simulink model "DFADAS2_SenFus_v1_201204RC_training_210115"  (R2018b)
settings: Solver=FixedStepDiscrete  StartTime=0.0  StopTime=inf  FixedStep=0.002  RelTol=1e-3  EnableMultiTasking=on
PreLoadFcn:
  | RTWConfigurationCB('preloadfcn', bdroot);
libraries: canmsglib x108, simulink x48, canfdmsglib x12
(part 19 of 28)

== system DFADAS2_SenFus_v1_201204RC_training_210115/Signal Input (Input)/Signal Input (50ms) (Input50)/Rear Right Radar(S1) Objects Information (RRRdr)/S0 Data Frame Read/Enabled Subsystem/M2ObjInfo/Subsystem1 ==
  const : Inport
  RemainderCnt : Inport  Port=2
  In : Inport  Port=3
  If : If  IfExpression=u1 >=0
  If Action Subsystem : Subsystem  TreatAsAtomicUnit=on
  If Action Subsystem1 : Subsystem  TreatAsAtomicUnit=on
  Merge : Merge
  Out : Outport
  wires:
  In/1 -> If Action Subsystem1/1(In1)
  const/1 -> If/1
  If/1 -> If Action Subsystem/Action
  If Action Subsystem1/1(Out1) -> Merge/2
  If/2 -> If Action Subsystem1/Action
  Merge/1 -> Out/1
  If Action Subsystem/1(Out1) -> Merge/1

== system DFADAS2_SenFus_v1_201204RC_training_210115/Signal Input (Input)/Signal Input (50ms) (Input50)/Rear Right Radar(S1) Objects Information (RRRdr)/S0 Data Frame Read/Enabled Subsystem/M3ObjInfo/If Action Subsystem1 ==
  msg : Inport
  "MValueSel " : Inport  Port=2
  obj_num : Inport  Port=3
  Action Port : ActionPort  ActionType=then
  Add : Sum
  Add2 : Sum
  Gain : Gain  Gain=48
  MValueSel : Constant  Value=24
  MValueSel2 : Constant  Value=[1:24]
  Product : Product
  Scope3 : Scope
  Selector : Selector  InputPortWidth=240  IndexOptions=Index vector (port)  Indices=[1 3]  OutputSizes=1
  Selector1 : Selector  InputPortWidth=240  IndexOptions=Index vector (port)  Indices=[1 3]  OutputSizes=1
  M30ObjInfo : Outport
  M31ObjInfo : Outport  Port=2
  wires:
  Product/1 -> M31ObjInfo/1
  obj_num/1 -> Scope3/1, Product/2
  Selector1/1 -> Product/1
  "MValueSel "/1 -> Gain/1
  Gain/1 -> Add2/1
  msg/1 -> Selector1/1, Selector/1
  Add/1 -> Selector1/2
  MValueSel/1 -> Add/2
  Add2/1 -> Selector/2, Add/1
  MValueSel2/1 -> Add2/2
  Selector/1 -> M30ObjInfo/1

== system DFADAS2_SenFus_v1_201204RC_training_210115/Signal Input (Input)/Signal Input (50ms) (Input50)/Rear Right Radar(S1) Objects Information (RRRdr)/S0 Data Frame Read/Enabled Subsystem/M3ObjInfo/If Action Subsystem2 ==
  Action Port : ActionPort  ActionType=elseif
  Constant : Constant  Value=[0 0 0 0 0 0 0 0 0 0 0 0 0 0 0 0 0 0 0 0 0 0 0 0]
  Constant1 : Constant  Value=[0 0 0 0 0 0 0 0 0 0 0 0 0 0 0 0 0 0 0 0 0 0 0 0]
  ZeroObjInfo0 : Outport
  ZeroObjInfo1 : Outport  Port=2
  wires:
  Constant/1 -> ZeroObjInfo0/1
  Constant1/1 -> ZeroObjInfo1/1

== system DFADAS2_SenFus_v1_201204RC_training_210115/Signal Input (Input)/Signal Input (50ms) (Input50)/Rear Right Radar(S1) Objects Information (RRRdr)/S0 Data Frame Read/Enabled Subsystem/M3ObjInfo/Subsystem1 ==
  const : Inport
  RemainderCnt : Inport  Port=2
  In : Inport  Port=3
  If : If  IfExpression=u1 >=0
  If Action Subsystem : Subsystem  TreatAsAtomicUnit=on
  If Action Subsystem1 : Subsystem  TreatAsAtomicUnit=on
  Merge : Merge
  Out : Outport
  wires:
  In/1 -> If Action Subsystem1/1(In1)
  const/1 -> If/1
  If/1 -> If Action Subsystem/Action
  If Action Subsystem1/1(Out1) -> Merge/2
  If/2 -> If Action Subsystem1/Action
  Merge/1 -> Out/1
  If Action Subsystem/1(Out1) -> Merge/1

== system DFADAS2_SenFus_v1_201204RC_training_210115/Signal Input (Input)/Signal Input (50ms) (Input50)/Rear Right Radar(S1) Objects Information (RRRdr)/S0 Data Frame Read/Enabled Subsystem/M4ObjInfo1/If Action Subsystem1 ==
  msg : Inport
  "MValueSel " : Inport  Port=2
  "obj_num " : Inport  Port=3
  Action Port : ActionPort  ActionType=then
  Add : Sum
  Add2 : Sum
  Gain : Gain  Gain=48
  MValueSel : Constant  Value=24
  MValueSel2 : Constant  Value=[1:24]
  Product : Product
  Scope3 : Scope
  Selector : Selector  InputPortWidth=240  IndexOptions=Index vector (port)  Indices=[1 3]  OutputSizes=1
  Selector1 : Selector  InputPortWidth=240  IndexOptions=Index vector (port)  Indices=[1 3]  OutputSizes=1
  M40ObjInfo : Outport
  M41ObjInfo : Outport  Port=2
  wires:
  Product/1 -> M41ObjInfo/1
  "obj_num "/1 -> Scope3/1, Product/2
  Selector1/1 -> Product/1
  Selector/1 -> M40ObjInfo/1
  MValueSel2/1 -> Add2/2
  Add2/1 -> Add/1, Selector/2
  MValueSel/1 -> Add/2
  Add/1 -> Selector1/2
  msg/1 -> Selector/1, Selector1/1
  Gain/1 -> Add2/1
  "MValueSel "/1 -> Gain/1

== system DFADAS2_SenFus_v1_201204RC_training_210115/Signal Input (Input)/Signal Input (50ms) (Input50)/Rear Right Radar(S1) Objects Information (RRRdr)/S0 Data Frame Read/Enabled Subsystem/M4ObjInfo1/If Action Subsystem2 ==
  Action Port : ActionPort  ActionType=elseif
  Constant : Constant  Value=[0 0 0 0 0 0 0 0 0 0 0 0 0 0 0 0 0 0 0 0 0 0 0 0]
  Constant1 : Constant  Value=[0 0 0 0 0 0 0 0 0 0 0 0 0 0 0 0 0 0 0 0 0 0 0 0]
  ZeroObjInfo0 : Outport
  ZeroObjInfo1 : Outport  Port=2
  wires:
  Constant1/1 -> ZeroObjInfo1/1
  Constant/1 -> ZeroObjInfo0/1

== system DFADAS2_SenFus_v1_201204RC_training_210115/Signal Input (Input)/Signal Input (50ms) (Input50)/Rear Right Radar(S1) Objects Information (RRRdr)/S0 Data Frame Read/Enabled Subsystem/M4ObjInfo1/Subsystem1 ==
  const : Inport
  RemainderCnt : Inport  Port=2
  In : Inport  Port=3
  If : If  IfExpression=u1 >=0
  If Action Subsystem : Subsystem  TreatAsAtomicUnit=on
  If Action Subsystem1 : Subsystem  TreatAsAtomicUnit=on
  Merge : Merge
  Out : Outport
  wires:
  In/1 -> If Action Subsystem1/1(In1)
  const/1 -> If/1
  If/1 -> If Action Subsystem/Action
  If Action Subsystem1/1(Out1) -> Merge/2
  If/2 -> If Action Subsystem1/Action
  Merge/1 -> Out/1
  If Action Subsystem/1(Out1) -> Merge/1

== system DFADAS2_SenFus_v1_201204RC_training_210115/Signal Input (Input)/Signal Input (50ms) (Input50)/Rear Right Radar(S1) Objects Information (RRRdr)/S0 Data Frame Read/Enabled Subsystem/Unpack/If Action Subsystem ==
  msg : Inport
  Action Port : ActionPort  ActionType=then
  Unpack : Subsystem
  RLRdrObjInfo : Outport
  MValue : Outport  Port=2
  wires:
  Unpack/1(RRRdrObjInfo) -> RLRdrObjInfo/1
  msg/1 -> Unpack/1(msg)
  Unpack/2(MValue) -> MValue/1

== system DFADAS2_SenFus_v1_201204RC_training_210115/Signal Input (Input)/Signal Input (50ms) (Input50)/Rear Right Radar(S1) Objects Information (RRRdr)/S0 Data Frame Read/Enabled Subsystem/Unpack/If Action Subsystem1 ==
  Action Port : ActionPort  ActionType=elseif
  Constant : Constant  Value=99
  DflMValue : Outport
  wires:
  Constant/1 -> DflMValue/1

== system DFADAS2_SenFus_v1_201204RC_training_210115/Signal Input (Input)/Signal Input (10ms) (Input10)/VehInfo/Body Electric System State Receive and Processing (BESRx)/Steering Lamp CAN Frame PreProcess (StLampCANFrmPPrcs)/CAN Diagnosis (CANDia)/CheckSum Diagnosis (ChkSumDia)/Bit Check(BChk) ==
  note: Bit Check Discription:
      | Byte0: Checksum
      | Byte1-7: Test signal
  BChk_bRawDa : Inport
  Bit Operating (BOp) : Subsystem
  Byte0 : Selector  IndexMode=Zero-based  InputPortWidth=8  IndexOptions=Index vector (dialog)  Indices=0  OutputSizes=1
  Byte1 : Selector  IndexMode=Zero-based  InputPortWidth=8  IndexOptions=Index vector (dialog)  Indices=1  OutputSizes=1
  Byte2 : Selector  IndexMode=Zero-based  InputPortWidth=8  IndexOptions=Index vector (dialog)  Indices=2  OutputSizes=1
  Byte3 : Selector  IndexMode=Zero-based  InputPortWidth=8  IndexOptions=Index vector (dialog)  Indices=3  OutputSizes=1
  Byte4 : Selector  IndexMode=Zero-based  InputPortWidth=8  IndexOptions=Index vector (dialog)  Indices=4  OutputSizes=1
  Byte5 : Selector  IndexMode=Zero-based  InputPortWidth=8  IndexOptions=Index vector (dialog)  Indices=5  OutputSizes=1
  Byte6 : Selector  IndexMode=Zero-based  InputPortWidth=8  IndexOptions=Index vector (dialog)  Indices=6  OutputSizes=1
  Byte7 : Selector  IndexMode=Zero-based  InputPortWidth=8  IndexOptions=Index vector (dialog)  Indices=7  OutputSizes=1
  BChk_efErrFlg : Outport
  wires:
  Byte0/1 -> Bit Operating (BOp)/1(BOp_bByte0)
  Bit Operating (BOp)/1(BOp_efChkSumErrFlg) -> BChk_efErrFlg/1
  Byte7/1 -> Bit Operating (BOp)/8(BOp_bByte7)
  Byte6/1 -> Bit Operating (BOp)/7(BOp_bByte6)
  Byte5/1 -> Bit Operating (BOp)/6(BOp_bByte5)
  Byte4/1 -> Bit Operating (BOp)/5(BOp_bByte4)
  Byte3/1 -> Bit Operating (BOp)/4(BOp_bByte3)
  Byte2/1 -> Bit Operating (BOp)/3(BOp_bByte2)
  Byte1/1 -> Bit Operating (BOp)/2(BOp_bByte1)
  BChk_bRawDa/1 -> Byte7/1, Byte6/1, Byte5/1, Byte4/1, Byte3/1, Byte2/1, Byte1/1, Byte0/1

== system DFADAS2_SenFus_v1_201204RC_training_210115/Signal Input (Input)/Signal Input (10ms) (Input10)/VehInfo/Function Keys State Receive and Processing (FKeyStRx)/Key Enable CAN Frame PreProcess (KeyEnaCANFrmPPrcs)/CAN Diagnosis (CANDia)/CheckSum Diagnosis (ChkSumDia)/Bit Check(BChk) ==
  note: Bit Check Discription:
      | Byte0: Checksum
      | Byte1-7: Test signal
  BChk_bRawDa : Inport
  Bit Operating (BOp) : Subsystem
  Byte0 : Selector  IndexMode=Zero-based  InputPortWidth=8  IndexOptions=Index vector (dialog)  Indices=0  OutputSizes=1
  Byte1 : Selector  IndexMode=Zero-based  InputPortWidth=8  IndexOptions=Index vector (dialog)  Indices=1  OutputSizes=1
  Byte2 : Selector  IndexMode=Zero-based  InputPortWidth=8  IndexOptions=Index vector (dialog)  Indices=2  OutputSizes=1
  Byte3 : Selector  IndexMode=Zero-based  InputPortWidth=8  IndexOptions=Index vector (dialog)  Indices=3  OutputSizes=1
  Byte4 : Selector  IndexMode=Zero-based  InputPortWidth=8  IndexOptions=Index vector (dialog)  Indices=4  OutputSizes=1
  Byte5 : Selector  IndexMode=Zero-based  InputPortWidth=8  IndexOptions=Index vector (dialog)  Indices=5  OutputSizes=1
  Byte6 : Selector  IndexMode=Zero-based  InputPortWidth=8  IndexOptions=Index vector (dialog)  Indices=6  OutputSizes=1
  Byte7 : Selector  IndexMode=Zero-based  InputPortWidth=8  IndexOptions=Index vector (dialog)  Indices=7  OutputSizes=1
  BChk_efErrFlg : Outport
  wires:
  BChk_bRawDa/1 -> Byte0/1, Byte1/1, Byte2/1, Byte3/1, Byte4/1, Byte5/1, Byte6/1, Byte7/1
  Byte1/1 -> Bit Operating (BOp)/2(BOp_bByte1)
  Byte2/1 -> Bit Operating (BOp)/3(BOp_bByte2)
  Byte3/1 -> Bit Operating (BOp)/4(BOp_bByte3)
  Byte4/1 -> Bit Operating (BOp)/5(BOp_bByte4)
  Byte5/1 -> Bit Operating (BOp)/6(BOp_bByte5)
  Byte6/1 -> Bit Operating (BOp)/7(BOp_bByte6)
  Byte7/1 -> Bit Operating (BOp)/8(BOp_bByte7)
  Bit Operating (BOp)/1(BOp_efChkSumErrFlg) -> BChk_efErrFlg/1
  Byte0/1 -> Bit Operating (BOp)/1(BOp_bByte0)

== system DFADAS2_SenFus_v1_201204RC_training_210115/Signal Input (Input)/Signal Input (10ms) (Input10)/VehInfo/MP5 Signal Receive (MP5Rx)1/CAN Diagnosis (CANDia)/CheckSum Diagnosis (ChkSumDia)/Bit Check(BChk)/Bit Operating (BOp) ==
  note: CheckSum Error Flag Discription:
      | 1 : Fault
      | 0 : Normal
  note: Checksum Preprocess -- ChksumPre
  Chksum in Frame : Inport
  BOp_bByte1 : Inport  Port=2
  BOp_bByte2 : Inport  Port=3
  BOp_bByte3 : Inport  Port=4
  BOp_bByte4 : Inport  Port=5
  BOp_bByte5 : Inport  Port=6
  BOp_bByte6 : Inport  Port=7
  BOp_bByte7 : Inport  Port=8
  Add : Sum  Inputs=+++++++
  Add1 : Sum  Inputs=+-
  Add2 : Sum  Inputs=+-
  ChksumPre1 : Subsystem
  ChksumPre2 : Subsystem
  ChksumPre3 : Subsystem
  ChksumPre4 : Subsystem
  ChksumPre5 : Subsystem
  ChksumPre6 : Subsystem
  ChksumPre7 : Subsystem
  Constant : Constant  Value=256  OutDataTypeStr=uint16  SampleTime=-1
  Constant1 : Constant  Value=255  OutDataTypeStr=uint8  SampleTime=-1
  Constant2 : Constant  OutDataTypeStr=uint8  SampleTime=-1
  Constant3 : Constant  Value=0  OutDataTypeStr=uint8  SampleTime=-1
  Data Type Conversion6 : DataTypeConversion  OutDataTypeStr=uint8
  Math Function : Math  Operator=mod  OutputSignalType=real  SaturateOnIntegerOverflow=on
  Switch : Switch  Criteria=u2 ~= 0
  BOp_efChkSumErrFlg : Outport
  wires:
  Switch/1 -> BOp_efChkSumErrFlg/1
  Constant3/1 -> Switch/3
  Constant2/1 -> Switch/1
  BOp_bByte7/1 -> ChksumPre7/1(In1)
  ChksumPre7/1(Out1) -> Add/7
  ChksumPre6/1(Out1) -> Add/6
  BOp_bByte6/1 -> ChksumPre6/2(In2)
  BOp_bByte5/1 -> ChksumPre6/1(In1)
  ChksumPre5/1(Out1) -> Add/5
  BOp_bByte4/1 -> ChksumPre5/2(In2)
  BOp_bByte3/1 -> ChksumPre5/1(In1)
  ChksumPre4/1(Out1) -> Add/4
  BOp_bByte2/1 -> ChksumPre4/1(In1), ChksumPre3/1(In1), ChksumPre2/1(In1)
  ChksumPre1/1(Out1) -> Add/1
  BOp_bByte1/1 -> ChksumPre1/1(In1)
  Constant1/1 -> Add1/1
  Math Function/1 -> Data Type Conversion6/1
  Constant/1 -> Math Function/2
  Add/1 -> Math Function/1
  Data Type Conversion6/1 -> Add1/2
  ChksumPre2/1(Out1) -> Add/2
  ChksumPre3/1(Out1) -> Add/3
  Chksum in Frame/1 -> Add2/1
  Add1/1 -> Add2/2
  Add2/1 -> Switch/2

== system DFADAS2_SenFus_v1_201204RC_training_210115/Signal Input (Input)/Signal Input (10ms) (Input10)/VehInfo/Vehicle Movement Signal Receive and Processing (VehMovRx)/VehSpd CAN Frame PreProcess (VehSpdCANFrmPPrcs)/CAN Diagnosis (CANDia)/CheckSum Diagnosis (ChkSumDia)/Bit Check(BChk) ==
  note: Bit Check Discription:
      | Byte0: Checksum
      | Byte1-7: Test signal
  BChk_bRawDa : Inport
  Bit Operating (BOp) : Subsystem
  Byte0 : Selector  IndexMode=Zero-based  InputPortWidth=8  IndexOptions=Index vector (dialog)  Indices=0  OutputSizes=1
  Byte1 : Selector  IndexMode=Zero-based  InputPortWidth=8  IndexOptions=Index vector (dialog)  Indices=1  OutputSizes=1
  Byte2 : Selector  IndexMode=Zero-based  InputPortWidth=8  IndexOptions=Index vector (dialog)  Indices=2  OutputSizes=1
  Byte3 : Selector  IndexMode=Zero-based  InputPortWidth=8  IndexOptions=Index vector (dialog)  Indices=3  OutputSizes=1
  Byte4 : Selector  IndexMode=Zero-based  InputPortWidth=8  IndexOptions=Index vector (dialog)  Indices=4  OutputSizes=1
  Byte5 : Selector  IndexMode=Zero-based  InputPortWidth=8  IndexOptions=Index vector (dialog)  Indices=5  OutputSizes=1
  Byte6 : Selector  IndexMode=Zero-based  InputPortWidth=8  IndexOptions=Index vector (dialog)  Indices=6  OutputSizes=1
  Byte7 : Selector  IndexMode=Zero-based  InputPortWidth=8  IndexOptions=Index vector (dialog)  Indices=7  OutputSizes=1
  BChk_efErrFlg : Outport
  wires:
  BChk_bRawDa/1 -> Byte0/1, Byte1/1, Byte2/1, Byte3/1, Byte4/1, Byte5/1, Byte6/1, Byte7/1
  Byte1/1 -> Bit Operating (BOp)/2(BOp_bByte1)
  Byte2/1 -> Bit Operating (BOp)/3(BOp_bByte2)
  Byte3/1 -> Bit Operating (BOp)/4(BOp_bByte3)
  Byte4/1 -> Bit Operating (BOp)/5(BOp_bByte4)
  Byte5/1 -> Bit Operating (BOp)/6(BOp_bByte5)
  Byte6/1 -> Bit Operating (BOp)/7(BOp_bByte6)
  Byte7/1 -> Bit Operating (BOp)/8(BOp_bByte7)
  Bit Operating (BOp)/1(BOp_efChkSumErrFlg) -> BChk_efErrFlg/1
  Byte0/1 -> Bit Operating (BOp)/1(BOp_bByte0)

== system DFADAS2_SenFus_v1_201204RC_training_210115/Signal Input (Input)/Signal Input (10ms) (Input10)/VehInfo/Vehicle Movement Signal Receive and Processing (VehMovRx)/Yaw State CAN Frame PreProcess (YawCANFrmPPrcs)/CAN Diagnosis (CANDia)/CheckSum Diagnosis (ChkSumDia)/Bit Check(BChk) ==
  note: Bit Check Discription:
      | Byte0: Checksum
      | Byte1-7: Test signal
  BChk_bRawDa : Inport
  Bit Operating (BOp) : Subsystem
  Byte0 : Selector  IndexMode=Zero-based  InputPortWidth=8  IndexOptions=Index vector (dialog)  Indices=0  OutputSizes=1
  Byte1 : Selector  IndexMode=Zero-based  InputPortWidth=8  IndexOptions=Index vector (dialog)  Indices=1  OutputSizes=1
  Byte2 : Selector  IndexMode=Zero-based  InputPortWidth=8  IndexOptions=Index vector (dialog)  Indices=2  OutputSizes=1
  Byte3 : Selector  IndexMode=Zero-based  InputPortWidth=8  IndexOptions=Index vector (dialog)  Indices=3  OutputSizes=1
  Byte4 : Selector  IndexMode=Zero-based  InputPortWidth=8  IndexOptions=Index vector (dialog)  Indices=4  OutputSizes=1
  Byte5 : Selector  IndexMode=Zero-based  InputPortWidth=8  IndexOptions=Index vector (dialog)  Indices=5  OutputSizes=1
  Byte6 : Selector  IndexMode=Zero-based  InputPortWidth=8  IndexOptions=Index vector (dialog)  Indices=6  OutputSizes=1
  Byte7 : Selector  IndexMode=Zero-based  InputPortWidth=8  IndexOptions=Index vector (dialog)  Indices=7  OutputSizes=1
  BChk_efErrFlg : Outport
  wires:
  BChk_bRawDa/1 -> Byte0/1, Byte1/1, Byte2/1, Byte3/1, Byte4/1, Byte5/1, Byte6/1, Byte7/1
  Byte1/1 -> Bit Operating (BOp)/2(BOp_bByte1)
  Byte2/1 -> Bit Operating (BOp)/3(BOp_bByte2)
  Byte3/1 -> Bit Operating (BOp)/4(BOp_bByte3)
  Byte4/1 -> Bit Operating (BOp)/5(BOp_bByte4)
  Byte5/1 -> Bit Operating (BOp)/6(BOp_bByte5)
  Byte6/1 -> Bit Operating (BOp)/7(BOp_bByte6)
  Byte7/1 -> Bit Operating (BOp)/8(BOp_bByte7)
  Bit Operating (BOp)/1(BOp_efChkSumErrFlg) -> BChk_efErrFlg/1
  Byte0/1 -> Bit Operating (BOp)/1(BOp_bByte0)

== system DFADAS2_SenFus_v1_201204RC_training_210115/Signal Input (Input)/Signal Input (50ms) (Input50)/Cmr/CmrInfo/L0 Information (L0Info) /CAN Diagnosis (CANDia)1/CheckSum Diagnosis (ChkSumDia)/Bit Check(BChk) ==
  note: Bit Check Discription:
      | Byte0: Checksum
      | Byte1-7: Test signal
  BChk_bRawDa : Inport
  Bit Operating (BOp) : Subsystem
  Byte0 : Selector  IndexMode=Zero-based  InputPortWidth=8  IndexOptions=Index vector (dialog)  Indices=0  OutputSizes=1
  Byte1 : Selector  IndexMode=Zero-based  InputPortWidth=8  IndexOptions=Index vector (dialog)  Indices=1  OutputSizes=1
  Byte2 : Selector  IndexMode=Zero-based  InputPortWidth=8  IndexOptions=Index vector (dialog)  Indices=2  OutputSizes=1
  Byte3 : Selector  IndexMode=Zero-based  InputPortWidth=8  IndexOptions=Index vector (dialog)  Indices=3  OutputSizes=1
  Byte4 : Selector  IndexMode=Zero-based  InputPortWidth=8  IndexOptions=Index vector (dialog)  Indices=4  OutputSizes=1
  Byte5 : Selector  IndexMode=Zero-based  InputPortWidth=8  IndexOptions=Index vector (dialog)  Indices=5  OutputSizes=1
  Byte6 : Selector  IndexMode=Zero-based  InputPortWidth=8  IndexOptions=Index vector (dialog)  Indices=6  OutputSizes=1
  Byte7 : Selector  IndexMode=Zero-based  InputPortWidth=8  IndexOptions=Index vector (dialog)  Indices=7  OutputSizes=1
  BChk_efErrFlg : Outport
  wires:
  BChk_bRawDa/1 -> Byte0/1, Byte1/1, Byte2/1, Byte3/1, Byte4/1, Byte5/1, Byte6/1, Byte7/1
  Byte1/1 -> Bit Operating (BOp)/2(BOp_bByte1)
  Byte2/1 -> Bit Operating (BOp)/3(BOp_bByte2)
  Byte3/1 -> Bit Operating (BOp)/4(BOp_bByte3)
  Byte4/1 -> Bit Operating (BOp)/5(BOp_bByte4)
  Byte5/1 -> Bit Operating (BOp)/6(BOp_bByte5)
  Byte6/1 -> Bit Operating (BOp)/7(BOp_bByte6)
  Byte7/1 -> Bit Operating (BOp)/8(BOp_bByte7)
  Bit Operating (BOp)/1(BOp_efChkSumErrFlg) -> BChk_efErrFlg/1
  Byte0/1 -> Bit Operating (BOp)/1(Chksum in Frame)

== system DFADAS2_SenFus_v1_201204RC_training_210115/Signal Input (Input)/Signal Input (50ms) (Input50)/Cmr/CmrInfo/L1 Information (L1Info)/CAN Diagnosis (CANDia)/CheckSum Diagnosis (ChkSumDia)/Bit Check(BChk) ==
  note: Bit Check Discription:
      | Byte0: Checksum
      | Byte1-7: Test signal
  BChk_bRawDa : Inport
  Bit Operating (BOp) : Subsystem
  Byte0 : Selector  IndexMode=Zero-based  InputPortWidth=8  IndexOptions=Index vector (dialog)  Indices=0  OutputSizes=1
  Byte1 : Selector  IndexMode=Zero-based  InputPortWidth=8  IndexOptions=Index vector (dialog)  Indices=1  OutputSizes=1
  Byte2 : Selector  IndexMode=Zero-based  InputPortWidth=8  IndexOptions=Index vector (dialog)  Indices=2  OutputSizes=1
  Byte3 : Selector  IndexMode=Zero-based  InputPortWidth=8  IndexOptions=Index vector (dialog)  Indices=3  OutputSizes=1
  Byte4 : Selector  IndexMode=Zero-based  InputPortWidth=8  IndexOptions=Index vector (dialog)  Indices=4  OutputSizes=1
  Byte5 : Selector  IndexMode=Zero-based  InputPortWidth=8  IndexOptions=Index vector (dialog)  Indices=5  OutputSizes=1
  Byte6 : Selector  IndexMode=Zero-based  InputPortWidth=8  IndexOptions=Index vector (dialog)  Indices=6  OutputSizes=1
  Byte7 : Selector  IndexMode=Zero-based  InputPortWidth=8  IndexOptions=Index vector (dialog)  Indices=7  OutputSizes=1
  BChk_efErrFlg : Outport
  wires:
  BChk_bRawDa/1 -> Byte0/1, Byte1/1, Byte2/1, Byte3/1, Byte4/1, Byte5/1, Byte6/1, Byte7/1
  Byte1/1 -> Bit Operating (BOp)/2(BOp_bByte1)
  Byte2/1 -> Bit Operating (BOp)/3(BOp_bByte2)
  Byte3/1 -> Bit Operating (BOp)/4(BOp_bByte3)
  Byte4/1 -> Bit Operating (BOp)/5(BOp_bByte4)
  Byte5/1 -> Bit Operating (BOp)/6(BOp_bByte5)
  Byte6/1 -> Bit Operating (BOp)/7(BOp_bByte6)
  Byte7/1 -> Bit Operating (BOp)/8(BOp_bByte7)
  Bit Operating (BOp)/1(BOp_efChkSumErrFlg) -> BChk_efErrFlg/1
  Byte0/1 -> Bit Operating (BOp)/1(Chksum in Frame)

== system DFADAS2_SenFus_v1_201204RC_training_210115/Signal Input (Input)/Signal Input (50ms) (Input50)/Cmr/CmrInfo/R0 Information (R0Info)/CAN Diagnosis (CANDia)/CheckSum Diagnosis (ChkSumDia)/Bit Check(BChk) ==
  note: Bit Check Discription:
      | Byte0: Checksum
      | Byte1-7: Test signal
  BChk_bRawDa : Inport
  Bit Operating (BOp) : Subsystem
  Byte0 : Selector  IndexMode=Zero-based  InputPortWidth=8  IndexOptions=Index vector (dialog)  Indices=0  OutputSizes=1
  Byte1 : Selector  IndexMode=Zero-based  InputPortWidth=8  IndexOptions=Index vector (dialog)  Indices=1  OutputSizes=1
  Byte2 : Selector  IndexMode=Zero-based  InputPortWidth=8  IndexOptions=Index vector (dialog)  Indices=2  OutputSizes=1
  Byte3 : Selector  IndexMode=Zero-based  InputPortWidth=8  IndexOptions=Index vector (dialog)  Indices=3  OutputSizes=1
  Byte4 : Selector  IndexMode=Zero-based  InputPortWidth=8  IndexOptions=Index vector (dialog)  Indices=4  OutputSizes=1
  Byte5 : Selector  IndexMode=Zero-based  InputPortWidth=8  IndexOptions=Index vector (dialog)  Indices=5  OutputSizes=1
  Byte6 : Selector  IndexMode=Zero-based  InputPortWidth=8  IndexOptions=Index vector (dialog)  Indices=6  OutputSizes=1
  Byte7 : Selector  IndexMode=Zero-based  InputPortWidth=8  IndexOptions=Index vector (dialog)  Indices=7  OutputSizes=1
  BChk_efErrFlg : Outport
  wires:
  BChk_bRawDa/1 -> Byte0/1, Byte1/1, Byte2/1, Byte3/1, Byte4/1, Byte5/1, Byte6/1, Byte7/1
  Byte1/1 -> Bit Operating (BOp)/2(BOp_bByte1)
  Byte2/1 -> Bit Operating (BOp)/3(BOp_bByte2)
  Byte3/1 -> Bit Operating (BOp)/4(BOp_bByte3)
  Byte4/1 -> Bit Operating (BOp)/5(BOp_bByte4)
  Byte5/1 -> Bit Operating (BOp)/6(BOp_bByte5)
  Byte6/1 -> Bit Operating (BOp)/7(BOp_bByte6)
  Byte7/1 -> Bit Operating (BOp)/8(BOp_bByte7)
  Bit Operating (BOp)/1(BOp_efChkSumErrFlg) -> BChk_efErrFlg/1
  Byte0/1 -> Bit Operating (BOp)/1(Chksum in Frame)

== system DFADAS2_SenFus_v1_201204RC_training_210115/Signal Input (Input)/Signal Input (50ms) (Input50)/Cmr/CmrInfo/R1 Information (R1Info)/CAN Diagnosis (CANDia)/CheckSum Diagnosis (ChkSumDia)/Bit Check(BChk) ==
  note: Bit Check Discription:
      | Byte0: Checksum
      | Byte1-7: Test signal
  BChk_bRawDa : Inport
  Bit Operating (BOp) : Subsystem
  Byte0 : Selector  IndexMode=Zero-based  InputPortWidth=8  IndexOptions=Index vector (dialog)  Indices=0  OutputSizes=1
  Byte1 : Selector  IndexMode=Zero-based  InputPortWidth=8  IndexOptions=Index vector (dialog)  Indices=1  OutputSizes=1
  Byte2 : Selector  IndexMode=Zero-based  InputPortWidth=8  IndexOptions=Index vector (dialog)  Indices=2  OutputSizes=1
  Byte3 : Selector  IndexMode=Zero-based  InputPortWidth=8  IndexOptions=Index vector (dialog)  Indices=3  OutputSizes=1
  Byte4 : Selector  IndexMode=Zero-based  InputPortWidth=8  IndexOptions=Index vector (dialog)  Indices=4  OutputSizes=1
  Byte5 : Selector  IndexMode=Zero-based  InputPortWidth=8  IndexOptions=Index vector (dialog)  Indices=5  OutputSizes=1
  Byte6 : Selector  IndexMode=Zero-based  InputPortWidth=8  IndexOptions=Index vector (dialog)  Indices=6  OutputSizes=1
  Byte7 : Selector  IndexMode=Zero-based  InputPortWidth=8  IndexOptions=Index vector (dialog)  Indices=7  OutputSizes=1
  BChk_efErrFlg : Outport
  wires:
  Byte0/1 -> Bit Operating (BOp)/1(Chksum in Frame)
  Bit Operating (BOp)/1(BOp_efChkSumErrFlg) -> BChk_efErrFlg/1
  Byte7/1 -> Bit Operating (BOp)/8(BOp_bByte7)
  Byte6/1 -> Bit Operating (BOp)/7(BOp_bByte6)
  Byte5/1 -> Bit Operating (BOp)/6(BOp_bByte5)
  Byte4/1 -> Bit Operating (BOp)/5(BOp_bByte4)
  Byte3/1 -> Bit Operating (BOp)/4(BOp_bByte3)
  Byte2/1 -> Bit Operating (BOp)/3(BOp_bByte2)
  Byte1/1 -> Bit Operating (BOp)/2(BOp_bByte1)
  BChk_bRawDa/1 -> Byte7/1, Byte6/1, Byte5/1, Byte4/1, Byte3/1, Byte2/1, Byte1/1, Byte0/1

== system DFADAS2_SenFus_v1_201204RC_training_210115/Signal Input (Input)/Signal Input (50ms) (Input50)/Front Left Radar(S2) Objects Information (FLRdr)/S0 Data Frame Read/Enabled Subsystem/M0ObjInfo/Subsystem1/If Action Subsystem ==
  Action Port : ActionPort  ActionType=then
  Constant : Constant  Value=0  OutDataTypeStr=uint16
  Out1 : Outport
  wires:
  Constant/1 -> Out1/1

== system DFADAS2_SenFus_v1_201204RC_training_210115/Signal Input (Input)/Signal Input (50ms) (Input50)/Front Left Radar(S2) Objects Information (FLRdr)/S0 Data Frame Read/Enabled Subsystem/M0ObjInfo/Subsystem1/If Action Subsystem1 ==
  In1 : Inport
  Action Port : ActionPort  ActionType=else
  Out1 : Outport
  wires:
  In1/1 -> Out1/1

== system DFADAS2_SenFus_v1_201204RC_training_210115/Signal Input (Input)/Signal Input (50ms) (Input50)/Front Left Radar(S2) Objects Information (FLRdr)/S0 Data Frame Read/Enabled Subsystem/M1ObjInfo1/Subsystem1/If Action Subsystem ==
  Action Port : ActionPort  ActionType=then
  Constant : Constant  Value=0  OutDataTypeStr=uint16
  Out1 : Outport
  wires:
  Constant/1 -> Out1/1

== system DFADAS2_SenFus_v1_201204RC_training_210115/Signal Input (Input)/Signal Input (50ms) (Input50)/Front Left Radar(S2) Objects Information (FLRdr)/S0 Data Frame Read/Enabled Subsystem/M1ObjInfo1/Subsystem1/If Action Subsystem1 ==
  In1 : Inport
  Action Port : ActionPort  ActionType=else
  Out1 : Outport
  wires:
  In1/1 -> Out1/1

== system DFADAS2_SenFus_v1_201204RC_training_210115/Signal Input (Input)/Signal Input (50ms) (Input50)/Front Left Radar(S2) Objects Information (FLRdr)/S0 Data Frame Read/Enabled Subsystem/M2ObjInfo/Subsystem1/If Action Subsystem ==
  Action Port : ActionPort  ActionType=then
  Constant : Constant  Value=0  OutDataTypeStr=uint16
  Out1 : Outport
  wires:
  Constant/1 -> Out1/1

== system DFADAS2_SenFus_v1_201204RC_training_210115/Signal Input (Input)/Signal Input (50ms) (Input50)/Front Left Radar(S2) Objects Information (FLRdr)/S0 Data Frame Read/Enabled Subsystem/M2ObjInfo/Subsystem1/If Action Subsystem1 ==
  In1 : Inport
  Action Port : ActionPort  ActionType=else
  Out1 : Outport
  wires:
  In1/1 -> Out1/1

== system DFADAS2_SenFus_v1_201204RC_training_210115/Signal Input (Input)/Signal Input (50ms) (Input50)/Front Left Radar(S2) Objects Information (FLRdr)/S0 Data Frame Read/Enabled Subsystem/M3ObjInfo/Subsystem1/If Action Subsystem ==
  Action Port : ActionPort  ActionType=then
  Constant : Constant  Value=0  OutDataTypeStr=uint16
  Out1 : Outport
  wires:
  Constant/1 -> Out1/1

== system DFADAS2_SenFus_v1_201204RC_training_210115/Signal Input (Input)/Signal Input (50ms) (Input50)/Front Left Radar(S2) Objects Information (FLRdr)/S0 Data Frame Read/Enabled Subsystem/M3ObjInfo/Subsystem1/If Action Subsystem1 ==
  In1 : Inport
  Action Port : ActionPort  ActionType=else
  Out1 : Outport
  wires:
  In1/1 -> Out1/1

== system DFADAS2_SenFus_v1_201204RC_training_210115/Signal Input (Input)/Signal Input (50ms) (Input50)/Front Left Radar(S2) Objects Information (FLRdr)/S0 Data Frame Read/Enabled Subsystem/M4ObjInfo1/Subsystem1/If Action Subsystem ==
  Action Port : ActionPort  ActionType=then
  Constant : Constant  Value=0  OutDataTypeStr=uint16
  Out1 : Outport
  wires:
  Constant/1 -> Out1/1

== system DFADAS2_SenFus_v1_201204RC_training_210115/Signal Input (Input)/Signal Input (50ms) (Input50)/Front Left Radar(S2) Objects Information (FLRdr)/S0 Data Frame Read/Enabled Subsystem/M4ObjInfo1/Subsystem1/If Action Subsystem1 ==
  In1 : Inport
  Action Port : ActionPort  ActionType=else
  Out1 : Outport
  wires:
  In1/1 -> Out1/1
